simulink model "assignment1_a"  (R2024b)
settings: Solver=VariableStepAuto  StartTime=0.0  StopTime=inf  RelTol=1e-3
settings Model: SnapshotInterval=5  PacingRate=224  Creator=ANURRADHA  LastModifiedBy=ANURRADHA

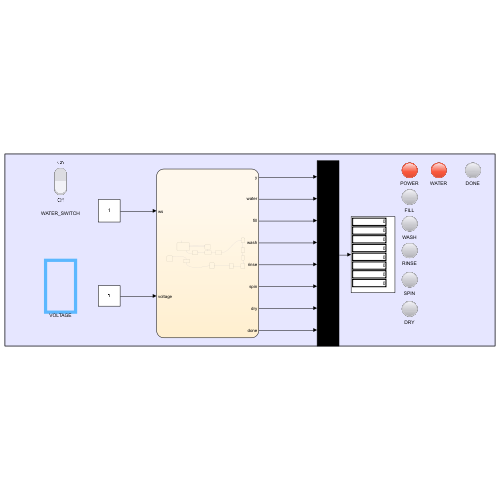
[thumbnail: Simulink's stored preview of the top-level diagram]
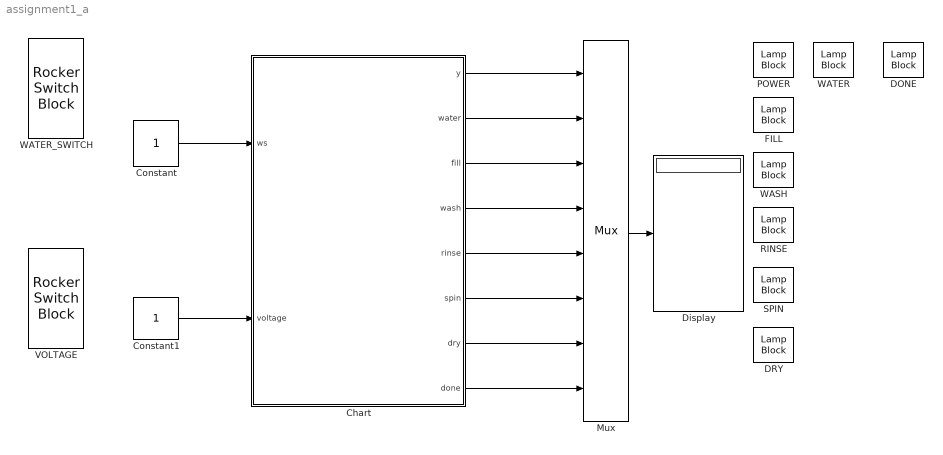
== system assignment1_a ==
  Chart : Stateflow chart  TreatAsAtomicUnit=on
  Constant : Constant
  Constant1 : Constant
  DONE : LampBlock  LabelPosition=Hide
  DRY : LampBlock  LabelPosition=Hide
  Display : Display
  FILL : LampBlock  LabelPosition=Hide
  Mux : Mux  Inputs=8
  POWER : LampBlock  LabelPosition=Hide
  RINSE : LampBlock  LabelPosition=Hide
  SPIN : LampBlock  LabelPosition=Hide
  VOLTAGE : RockerSwitchBlock  LabelPosition=Hide
      settings: Values={{'Off', 'On'}, [0 1]}
  WASH : LampBlock  LabelPosition=Hide
  WATER : LampBlock  LabelPosition=Hide
  WATER_SWITCH : RockerSwitchBlock  LabelPosition=Hide
      settings: Values={{'Off', 'On'}, [0 1]}
  wires:
  Constant1/1 -> Chart/2(voltage)
  Constant/1 -> Chart/1(ws)
  Chart/4(wash) -> Mux/4
  Chart/3(fill) -> Mux/3
  Chart/2(water) -> Mux/2
  Chart/6(spin) -> Mux/6
  Chart/5(rinse) -> Mux/5
  Chart/1(y) -> Mux/1
  Chart/8(done) -> Mux/8
  Mux/1 -> Display/1
  Chart/7(dry) -> Mux/7

== stateflow chart assignment1_a/Chart ==
  state FILL
    entry:
    fill=1;
    exit:
    fill=0;
  state power_off
    entry:
    y=0;
    exit:
    y=1
  state power_on
    entry:
    y=1;
    exit:
    y=0;
  state WASH
    entry:
    wash=1;
    exit:
    wash=0;
  state water_high
    water=1;
  state water_check
    y=1;
  state water_low
    water=0;
  state RINSE
    entry:
    rinse=1;
    exit:
    rinse=0;
  state POWER_OFF
    entry:
    y=0;
    during:
    done=0;
  state water_low1
    water=0;
  state DONE_
    done=1;
  state DRY
    entry:
    dry=1;
    exit:
    dry=0;
  state SPIN
    entry:
    spin=1;
    exit:
    spin=0;
  water_high -> FILL : after(100,sec)
  (default) -> power_off
  FILL -> WASH : after(500,sec)
  power_off -> power_on : [voltage==1]
  power_on -> power_off [order 1] : [voltage==0]
  power_on -> water_check [order 2]
  water_low -> power_off
  water_check -> water_high [order 1] : [ws>=1]
  water_check -> water_low [order 2] : [ws==0]
  WASH -> RINSE : after(200,sec)
  water_low1 -> POWER_OFF : after (200,sec)
  RINSE -> SPIN : after(300,sec)
  DONE_ -> water_low1
  DRY -> DONE_ : after(450,sec)
  SPIN -> DRY : after(400,sec)
  data: y output; water output; fill output; wash output; ws input; voltage input; rinse output; spin output; dry output; done output
